simulink model "AMR_odometria_udp_lidarloc_24a"  (R2024a)
settings: configuration reference "SharedConfig" (kept outside this file)
undefined symbols (not defined in the file): udp_odometry_header_version, udp_odometry_magic_word, udp_odometry_msg_type, udp_odometry_msg_type_version, udp_odometry_payload_length, udp_odometry_payload_type
libraries: slrealtimeutilitieslib x5
settings Model: DataDictionary=configuration_dictionary.sldd  Creator=matlab.cut  LastModifiedBy=matlab.cut
settings ConfigSetRef: SourceName=SharedConfig

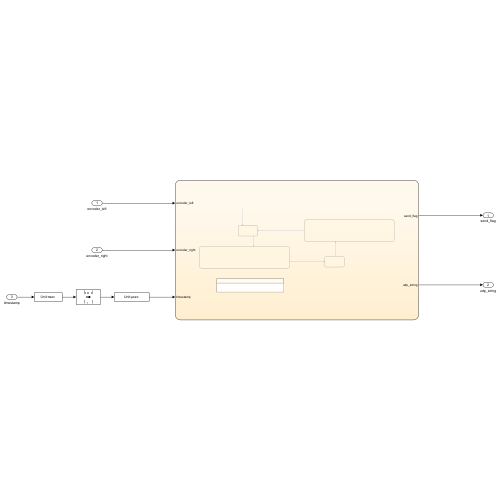
[thumbnail: Simulink's stored preview of the top-level diagram]
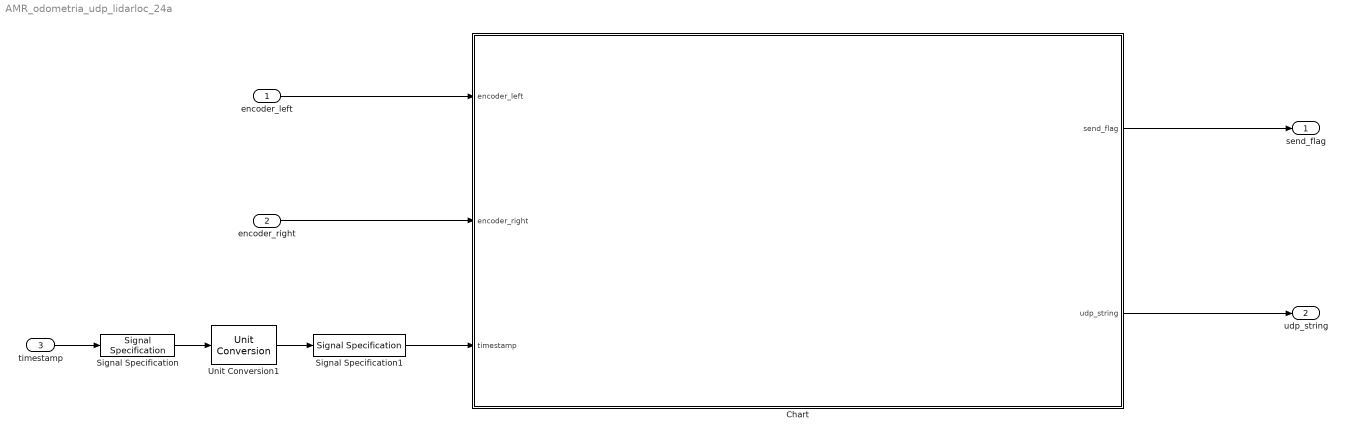
== system AMR_odometria_udp_lidarloc_24a ==
  encoder_left : Inport  OutDataTypeStr=int64
  encoder_right : Inport  Port=2  OutDataTypeStr=int64
  timestamp : Inport  Port=3  OutDataTypeStr=uint64
  Chart : Stateflow chart  TreatAsAtomicUnit=on
  Signal Specification : SignalSpecification  Unit=nsec
  Signal Specification1 : SignalSpecification  Unit=µsec
  Unit Conversion1 : UnitConversion  OutputType=Inherit: Inherit via back propagation
  send_flag : Outport
  udp_string : Outport  Port=2  OutDataTypeStr=uint8  PortDimensions=40
  wires:
  encoder_left/1 -> Chart/1(encoder_left)
  Chart/1(send_flag) -> send_flag/1
  encoder_right/1 -> Chart/2(encoder_right)
  Chart/2(udp_string) -> udp_string/1
  Unit Conversion1/1 -> Signal Specification1/1
  Signal Specification/1 -> Unit Conversion1/1
  timestamp/1 -> Signal Specification/1
  Signal Specification1/1 -> Chart/3(timestamp)

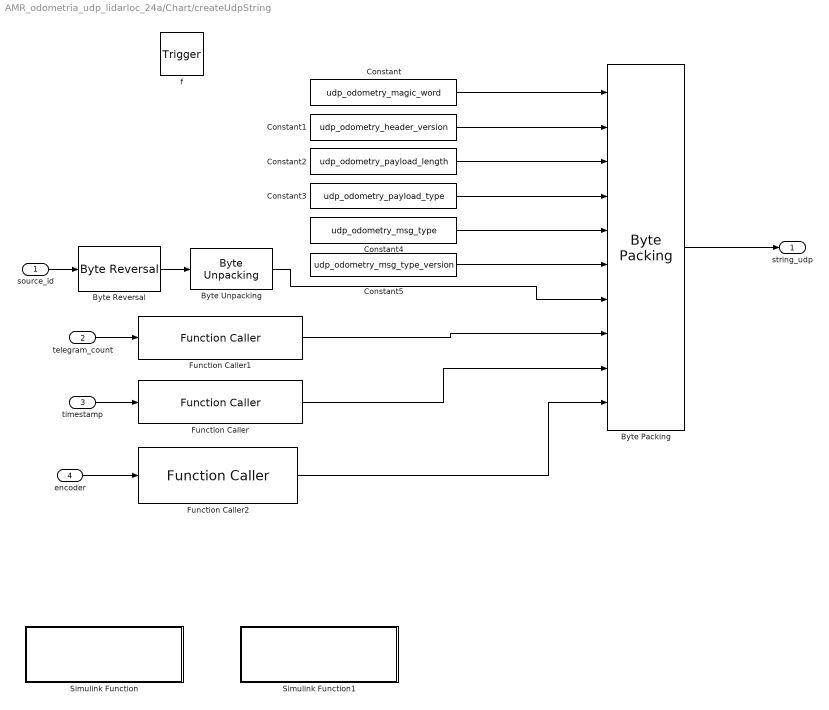
== system AMR_odometria_udp_lidarloc_24a/Chart/createUdpString ==
  source_id : Inport  OutDataTypeStr=uint16  PortDimensions=1
  telegram_count : Inport  Port=2  OutDataTypeStr=uint64  PortDimensions=1
  timestamp : Inport  Port=3  OutDataTypeStr=uint64  PortDimensions=1
  encoder : Inport  Port=4  OutDataTypeStr=int64  PortDimensions=1
  f : TriggerPort  TriggerType=function-call  VariantControl=(inherit)
      settings: CopyFcn=Stateflow.SLINSF.SimulinkMan.removeBlockPreDeleteFcn  PreDeleteFcn=Stateflow.SLINSF.SimulinkMan.unsafePredeleteFcn
  Byte Packing : slrealtimeutilitieslib/Byte Packing  MaskPackedDataType=uint8  MaskUnpackedDataTypes={['uint8'],['uint8'],['uint8'],['uint8'],['uint8'],['uint8'],['uint8'],['uint8'],['uint8'],['uint8']}  MaskAlignment=1
  Byte Reversal : slrealtimeutilitieslib/Byte Reversal  numInp=1
  Byte Unpacking : slrealtimeutilitieslib/Byte Unpacking  MaskUnpackedDataTypes={'uint8'}  MaskUnpackedDataSizes={[2]}  MaskAlignment=1
  Constant : Constant  Value=udp_odometry_magic_word
  Constant1 : Constant  Value=udp_odometry_header_version
  Constant2 : Constant  Value=udp_odometry_payload_length
  Constant3 : Constant  Value=udp_odometry_payload_type
  Constant4 : Constant  Value=udp_odometry_msg_type
  Constant5 : Constant  Value=udp_odometry_msg_type_version
  Function Caller : FunctionCaller  FunctionPrototype=y = invertBytesUint64(u)  InputArgumentSpecifications=<Enter example>  OutputArgumentSpecifications=<Enter example>
  Function Caller1 : FunctionCaller  FunctionPrototype=y = invertBytesUint64(u)  InputArgumentSpecifications=<Enter example>  OutputArgumentSpecifications=<Enter example>
  Function Caller2 : FunctionCaller  FunctionPrototype=y = invertBytesInt64(u)  InputArgumentSpecifications=<Enter example>  OutputArgumentSpecifications=<Enter example>
  Simulink Function : Subsystem  TreatAsAtomicUnit=on
  Simulink Function1 : Subsystem  TreatAsAtomicUnit=on
  string_udp : Outport  OutDataTypeStr=uint8  PortDimensions=40
  wires:
  Constant/1 -> Byte Packing/1
  Constant1/1 -> Byte Packing/2
  Constant2/1 -> Byte Packing/3
  Constant3/1 -> Byte Packing/4
  Constant4/1 -> Byte Packing/5
  Constant5/1 -> Byte Packing/6
  source_id/1 -> Byte Reversal/1
  encoder/1 -> Function Caller2/1
  Byte Packing/1 -> string_udp/1
  Byte Reversal/1 -> Byte Unpacking/1
  Byte Unpacking/1 -> Byte Packing/7
  Function Caller2/1 -> Byte Packing/10
  timestamp/1 -> Function Caller/1
  Function Caller/1 -> Byte Packing/9
  telegram_count/1 -> Function Caller1/1
  Function Caller1/1 -> Byte Packing/8

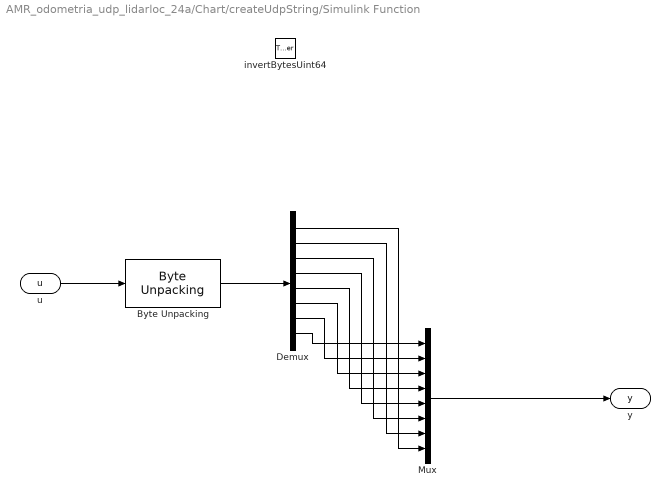
== system AMR_odometria_udp_lidarloc_24a/Chart/createUdpString/Simulink Function ==
  invertBytesUint64 : TriggerPort  TriggerType=function-call  IsSimulinkFunction=on  FunctionName=invertBytesUint64  FunctionVisibility=scoped  VariantControl=(inherit)
  Byte Unpacking : slrealtimeutilitieslib/Byte Unpacking  MaskUnpackedDataTypes={['uint8']}  MaskUnpackedDataSizes={[8]}  MaskAlignment=1
  Demux : Demux  Outputs=8
  Mux : Mux  Inputs=8
  u : ArgIn  DisableCoverage=on  OutDataTypeStr=uint64  ArgumentName=u
  y : ArgOut  DisableCoverage=on  OutDataTypeStr=uint8  PortDimensions=8  ArgumentName=y
  wires:
  Demux/5 -> Mux/4
  Demux/4 -> Mux/5
  Demux/8 -> Mux/1
  Byte Unpacking/1 -> Demux/1
  Demux/3 -> Mux/6
  Demux/1 -> Mux/8
  Demux/2 -> Mux/7
  Demux/6 -> Mux/3
  Demux/7 -> Mux/2
  Mux/1 -> y/1
  u/1 -> Byte Unpacking/1

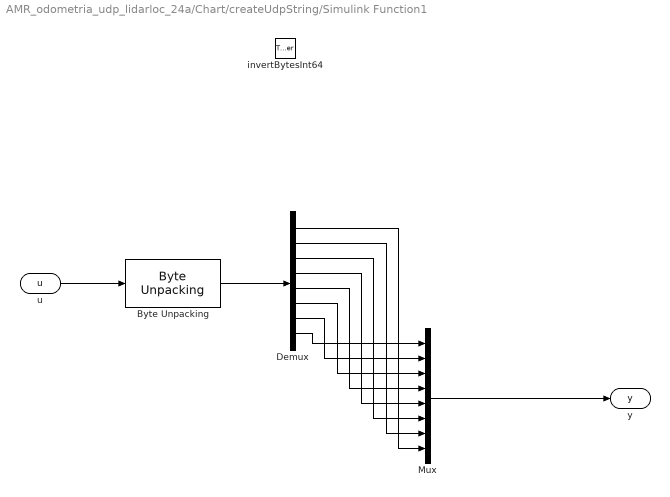
== system AMR_odometria_udp_lidarloc_24a/Chart/createUdpString/Simulink Function1 ==
  invertBytesInt64 : TriggerPort  TriggerType=function-call  IsSimulinkFunction=on  FunctionName=invertBytesInt64  FunctionVisibility=scoped  VariantControl=(inherit)
  Byte Unpacking : slrealtimeutilitieslib/Byte Unpacking  MaskUnpackedDataTypes={['uint8']}  MaskUnpackedDataSizes={[8]}  MaskAlignment=1
  Demux : Demux  Outputs=8
  Mux : Mux  Inputs=8
  u : ArgIn  DisableCoverage=on  OutDataTypeStr=int64  ArgumentName=u
  y : ArgOut  DisableCoverage=on  OutDataTypeStr=uint8  PortDimensions=8  ArgumentName=y
  wires:
  Demux/5 -> Mux/4
  Demux/4 -> Mux/5
  Demux/8 -> Mux/1
  Byte Unpacking/1 -> Demux/1
  Demux/3 -> Mux/6
  Demux/1 -> Mux/8
  Demux/2 -> Mux/7
  Demux/6 -> Mux/3
  Demux/7 -> Mux/2
  Mux/1 -> y/1
  u/1 -> Byte Unpacking/1

== stateflow chart AMR_odometria_udp_lidarloc_24a/Chart ==
  state send_right
    entry:
    j = j + 1;
    source_id = 22;
    telegram_count = j;
    udp_string = createUdpString(source_id, telegram_count, timestamp, encoder_right);
    exit:
    send_flag = true;
  state idle
    exit:
    send_flag = false;
  state send_left
    entry:
    i = i + 1;
    source_id = 21;
    telegram_count = i;
    udp_string = createUdpString(source_id, telegram_count, timestamp, encoder_left);
    exit:
    send_flag = true;
  state idle_udp_interval
    exit:
    send_flag = false;
  state string_udp = createUdpString(source_id,telegram_count,timestamp,encoder) [function]
  (default) -> idle : {i=0; j=0;}
  send_right -> idle : after(1,msec)
  idle -> send_left : after(24, msec)
  idle_udp_interval -> send_right : after(4,msec)
  send_left -> idle_udp_interval : after(1,msec)
  data: source_id function_input uint16 size=1; telegram_count function_input uint64 size=1; timestamp function_input uint64 size=1; encoder function_input int64 size=1; string_udp function_output uint8 size=40; encoder_left input int64; send_flag output; encoder_right input int64; udp_string output; i local uint64; j local uint64; timestamp input uint64; source_id local uint16; telegram_count local uint64
